simulink model "GFLIB_ControllerPIr_BAM_F16"  (Simulink 7.3)
settings: Solver=ode45  StartTime=0.0  StopTime=10.0  RelTol=1e-3
undefined symbols (not defined in the file): f16CC1, f16CC2, u16NShift
settings Model: Creator=RE004C  LastModifiedBy=RE004C
settings HardwareCC: ProdIntDivRoundTo=Zero  ProdEndianess=BigEndian  ProdHWDeviceType=Freescale->32-bit PowerPC

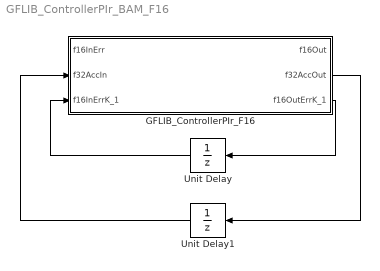
== system GFLIB_ControllerPIr_BAM_F16 ==
  GFLIB_ControllerPIr_F16 : Subsystem  mask(GFLIB_ControllerPIr_F16){f16CC1=f16CC1, f16CC2=f16CC2, u16NShift=u16NShift}
      mask help: Bit accurate model of reccurent form PI controller. All parameters as well as input and output are 16-bit integers except for u16NShift parameter which is 16-bit unsigned integer.
      mask init:
      | pos = get_param(gcb, 'Position');width = pos(3) - pos(1); height = pos(4) - pos(2);tX=width/2;tY=height*0.9;
      mask Display:
      | color('black');
      | port_label('input',1,'f16InErr');
      | port_label('input',2,'f32AccIn');
      | port_label('input',3,'f16InErrK_1');
      | port_label('output',1,'f16Out');
      | port_label('output',2,'f32AccOut');
      | port_label('output',3,'f16OutErrK_1');
      | color('black');
      | disp('GFLIB_ControllerPIr_F16');
      | color('blue');
      | text(tX,tY, 'BAM', 'horizontalAlignment', 'center');
  Unit Delay : UnitDelay  SampleTime=-1
  Unit Delay1 : UnitDelay  SampleTime=-1
  wires:
  GFLIB_ControllerPIr_F16/3(f16OutErrK_1) -> Unit Delay/1
  Unit Delay/1 -> GFLIB_ControllerPIr_F16/3(f16InErrK_1)
  GFLIB_ControllerPIr_F16/2(f32AccOut) -> Unit Delay1/1
  Unit Delay1/1 -> GFLIB_ControllerPIr_F16/2(f32AccIn)

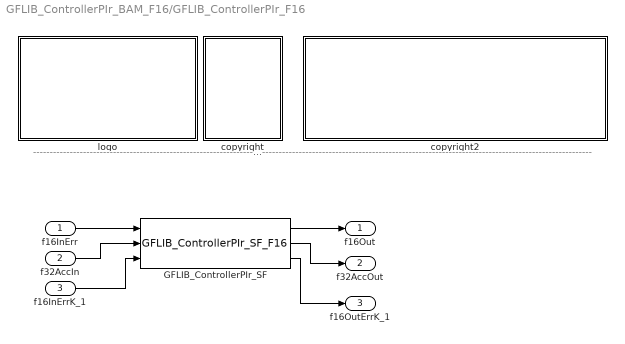
== system GFLIB_ControllerPIr_BAM_F16/GFLIB_ControllerPIr_F16 ==
  note: ---------------------------------------------------------------------------------------------------------------------------------------------------------------------------------------------------
  f16InErr : Inport  OutDataType=fixdt(1, 16)  OutScaling=2^0
  f32AccIn : Inport  Port=2  OutDataType=fixdt(1, 16)  OutScaling=2^0
  f16InErrK_1 : Inport  Port=3  OutDataType=fixdt(1, 16)  OutScaling=2^0
  GFLIB_ControllerPIr_SF : S-Function  FunctionName=GFLIB_ControllerPIr_SF_F16  Parameters=f16CC1,f16CC2,u16NShift  EnableBusSupport=off
  copyright : Subsystem
      mask Display: text(10,90,'FILE:');text(10,75,'DESRIPTION:')text(10,60,'COPYRIGHT:')text(10,45,'VERSION:')text(10,30,'DATE:')
  copyright2 : Subsystem
      mask Display: text(10,90,'GFLIB_ControllerPIr_BAM_F16.mdl');text(10,75,'Recurrent form of a standard PI controller without implemented anti-windup.');text(10,60,'Freescale')text(10,45,'0.1');text(10,30,'20-Jan-2012');
  logo : Subsystem
      mask Display: image(imread('logo.jpg'))
  f16Out : Outport  OutDataType=fixdt(1, 16)  OutScaling=2^0
  f32AccOut : Outport  Port=2  OutDataType=fixdt(1, 16)  OutScaling=2^0
  f16OutErrK_1 : Outport  Port=3  OutDataType=fixdt(1, 16)  OutScaling=2^0
  wires:
  f16InErr/1 -> GFLIB_ControllerPIr_SF/1
  GFLIB_ControllerPIr_SF/1 -> f16Out/1
  f32AccIn/1 -> GFLIB_ControllerPIr_SF/2
  f16InErrK_1/1 -> GFLIB_ControllerPIr_SF/3
  GFLIB_ControllerPIr_SF/2 -> f32AccOut/1
  GFLIB_ControllerPIr_SF/3 -> f16OutErrK_1/1

== system GFLIB_ControllerPIr_BAM_F16/GFLIB_ControllerPIr_F16/copyright ==

== system GFLIB_ControllerPIr_BAM_F16/GFLIB_ControllerPIr_F16/copyright2 ==

== system GFLIB_ControllerPIr_BAM_F16/GFLIB_ControllerPIr_F16/logo ==
